simulink model "Estimators"  (R2018a)
settings: Solver=VariableStepAuto  StartTime=0.0  StopTime=10.0  RelTol=1e-3
PreLoadFcn:
  | modelDir = fileparts(get_param(bdroot, 'FileName'));
  | addpath(fullfile(modelDir));
  | addpath(fullfile(modelDir,'../../Parameters'));
  | addpath(fullfile(modelDir,'../../Misc'));
  | 
  | Parameters_Estimators
  | Parameters_Simulation
InitFcn:
  | Parameters_Estimators
  | Parameters_Simulation
undefined symbols (not defined in the file or in its folder): Ts, UseMadgwick
settings Model: Creator=Thomas  LastModifiedBy=Thomas

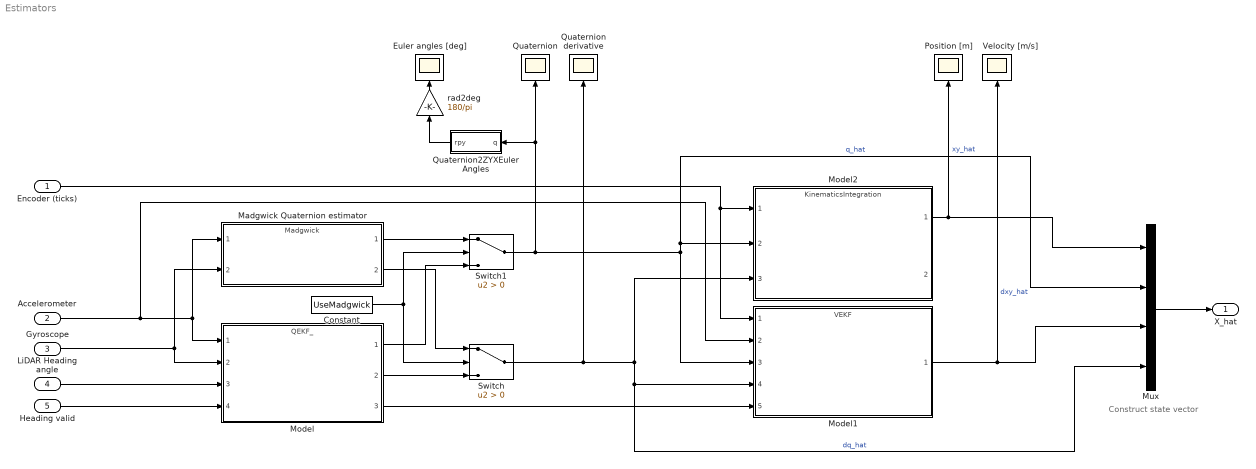
== system Estimators ==
  note: Construct state vector
  Encoder (ticks) : Inport
  Accelerometer : Inport  Port=2
  Gyroscope : Inport  Port=3
  LiDAR Heading angle : Inport  Port=4
  Heading valid : Inport  Port=5
  Constant : Constant  Value=UseMadgwick
  Euler angles [deg] : Scope
  Madgwick Quaternion estimator : ModelReference  ModelNameDialog=Madgwick  SimulationMode=Normal  ModelReferenceVersion=1.8
  Model : ModelReference  ModelNameDialog=QEKF_  SimulationMode=Normal  ModelReferenceVersion=1.28
  Model1 : ModelReference  ModelNameDialog=VEKF  SimulationMode=Normal  ModelReferenceVersion=1.29
  Model2 : ModelReference  ModelNameDialog=KinematicsIntegration  SimulationMode=Normal  ModelReferenceVersion=1.9
  Mux : Mux
  Position [m] : Scope
  Quaternion : Scope
  Quaternion derivative : Scope
  Quaternion2ZYXEulerAngles : MATLAB Function  TreatAsAtomicUnit=on
  Switch : Switch  Criteria=u2 > Threshold
  Switch1 : Switch  Criteria=u2 > Threshold
  Velocity [m/s] : Scope
  rad2deg : Gain  Gain=180/pi
  X_hat : Outport  SampleTime=Ts
  wires:
  LiDAR Heading angle/1 -> Model/3
  Heading valid/1 -> Model/4
  Accelerometer/1 -> Model1/2, Model/1, Madgwick Quaternion estimator/1
  Gyroscope/1 -> Model/2, Madgwick Quaternion estimator/2
  Mux/1 -> X_hat/1
  Constant/1 -> Switch/2, Switch1/2
  Madgwick Quaternion estimator/1 -> Switch1/1
  Model/2 -> Switch/3
  Model/1 -> Switch1/3
  Madgwick Quaternion estimator/2 -> Switch/1
  Switch1/1 -> Mux/2, Model2/2, Model1/3, Quaternion/1, Quaternion2ZYXEulerAngles/1(q)  "q_hat"
  Switch/1 -> Mux/4, Model1/4, Model2/3, Quaternion derivative/1  "dq_hat"
  Model/3 -> Model1/5
  Encoder (ticks)/1 -> Model1/1, Model2/1
  Model2/1 -> Mux/1, Position [m]/1  "xy_hat"
  Model1/1 -> Velocity [m/s]/1, Mux/3  "dxy_hat"
  Quaternion2ZYXEulerAngles/1(rpy) -> rad2deg/1
  rad2deg/1 -> Euler angles [deg]/1

== matlab function Estimators/Quaternion2ZYXEulerAngles ==
  data: q input; rpy output
function rpy = Quaternion2ZYXEulerAngles(q)
    rpy = Quaternion2ZYXEulerAngles(q);
end
